simulink library "uavsimBlockset_ZagiUAS_externalForces"  (Simulink 8.0)
settings: Solver=ode45  StartTime=0.0  StopTime=10.0  RelTol=1e-3
libraries: uavsimBlockset_ServoHS55 x4, uavsimBlockset_Zagi_Aerandpropulsion x1, uavsimblockset_SixDOFKinematics x1
settings Model: Creator=mstolle  LastModifiedBy=j.bolting

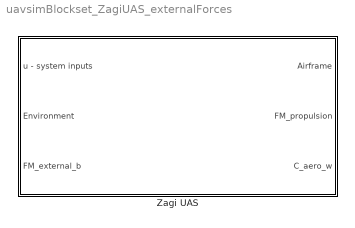
== system uavsimBlockset_ZagiUAS_externalForces ==
  Zagi UAS : Subsystem  mask{mask_zagi_phithetapsi0=[0 0 0]', mask_zagi_p0_ECEF_lla=[0 0 50]', mask_zagi_pqr0=[0 0 0]', mask_zagi_uvw0=[30 0 0]}
      mask prompts: mask_zagi_phithetapsi0 "Initial euler angles [rad]"; mask_zagi_p0_ECEF_lla "Initial position ECEF [rad rad m]"; mask_zagi_pqr0 "Initial body rotation rates [rad/s]"; mask_zagi_uvw0 "Initial velocity body frame [m/s]"
      mask Display: image(imread('images/zagi_slope.png'),[.3, .3, .4, .4])

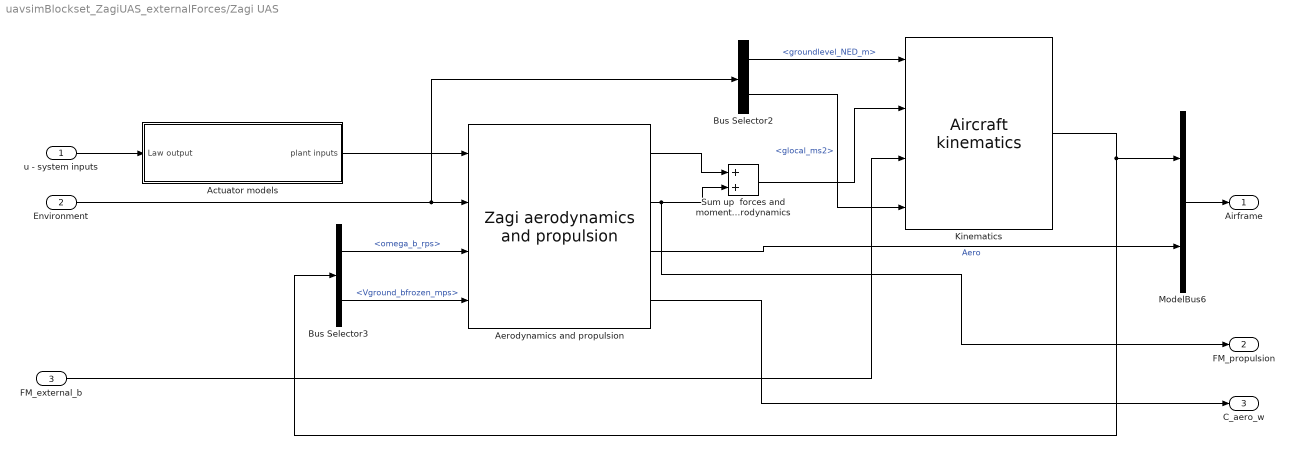
== system uavsimBlockset_ZagiUAS_externalForces/Zagi UAS ==
  u - system inputs : Inport  OutDataTypeStr=Bus: CMD
  Environment : Inport  Port=2  OutDataTypeStr=Bus: Environment
  FM_external_b : Inport  Port=3
  Actuator models : Subsystem
  Aerodynamics and propulsion : uavsimBlockset_Zagi_Aerandpropulsion/Zagi aerodynamics and propulsion  SystemSampleTime=-1
  Bus Selector2 : BusSelector  OutputSignals=groundlevel_NED_m,glocal_ms2
  Bus Selector3 : BusSelector  OutputSignals=RotationalVelocity.omega_b_rps,Velocity.Vground_bfrozen_mps
  Kinematics : uavsimblockset_SixDOFKinematics/Aircraft kinematics  mask_inertia=uavsim.zagi.inertiaTensor  mask_mass=uavsim.zagi.mass  mask_P0_ECEF_lla=mask_zagi_p0_ECEF_lla  mask_uvw0=mask_zagi_uvw0  mask_phithetapsi0=mask_zagi_phithetapsi0  mask_omega0=mask_zagi_pqr0
  ModelBus6 : BusCreator  Inputs=2  OutDataTypeStr=Bus: Airframe  NonVirtualBus=on
  Sum up  forces and moments of engine and aircraft aerodynamics : Sum
  Airframe : Outport  OutDataTypeStr=Bus: Airframe
  FM_propulsion : Outport  Port=2
  C_aero_w : Outport  Port=3
  wires:
  Kinematics/1 -> Bus Selector3/1, ModelBus6/1
  Bus Selector2/1 -> Kinematics/1  "<groundlevel_NED_m>"
  Bus Selector2/2 -> Kinematics/4  "<glocal_ms2>"
  u - system inputs/1 -> Actuator models/1(Law output)
  Bus Selector3/1 -> Aerodynamics and propulsion/3  "<omega_b_rps>"
  Bus Selector3/2 -> Aerodynamics and propulsion/4  "<Vground_bfrozen_mps>"
  ModelBus6/1 -> Airframe/1
  Aerodynamics and propulsion/3 -> ModelBus6/2  "Aero"
  Environment/1 -> Bus Selector2/1, Aerodynamics and propulsion/2
  Actuator models/1(plant inputs) -> Aerodynamics and propulsion/1
  FM_external_b/1 -> Kinematics/3
  Aerodynamics and propulsion/4 -> C_aero_w/1
  Aerodynamics and propulsion/1 -> Sum up  forces and moments of engine and aircraft aerodynamics/1
  Aerodynamics and propulsion/2 -> FM_propulsion/1, Sum up  forces and moments of engine and aircraft aerodynamics/2
  Sum up  forces and moments of engine and aircraft aerodynamics/1 -> Kinematics/2

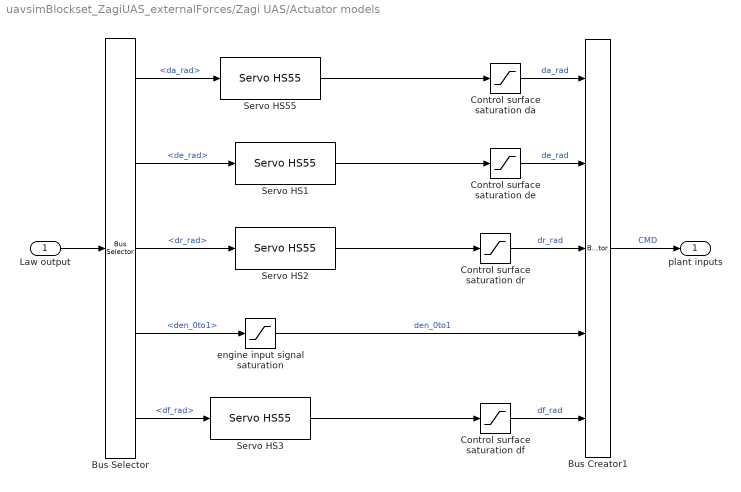
== system uavsimBlockset_ZagiUAS_externalForces/Zagi UAS/Actuator models ==
  Law output : Inport  OutDataTypeStr=Bus: CMD
  Bus Creator1 : BusCreator  Inputs=5  OutDataTypeStr=Bus: CMD  NonVirtualBus=on
  Bus Selector : BusSelector  OutputSignals=da_rad,de_rad,dr_rad,den_0to1,df_rad
  Control surface saturation da : Saturate  UpperLimit=deg2rad(45)  LowerLimit=deg2rad(-45)
  Control surface saturation de : Saturate  UpperLimit=deg2rad(45)  LowerLimit=deg2rad(-45)
  Control surface saturation df : Saturate  UpperLimit=deg2rad(45)  LowerLimit=deg2rad(-45)
  Control surface saturation dr : Saturate  UpperLimit=deg2rad(45)  LowerLimit=deg2rad(-45)
  Servo HS{1..3,55} (4 alike) : uavsimBlockset_ServoHS55/Servo HS55
  engine input signal saturation : Saturate  UpperLimit=1  LowerLimit=0
  plant inputs : Outport  OutDataTypeStr=Bus: CMD
  wires:
  Servo HS2/1 -> Control surface saturation dr/1
  Servo HS1/1 -> Control surface saturation de/1
  Servo HS55/1 -> Control surface saturation da/1
  Control surface saturation da/1 -> Bus Creator1/1  "da_rad"
  Control surface saturation de/1 -> Bus Creator1/2  "de_rad"
  Control surface saturation dr/1 -> Bus Creator1/3  "dr_rad"
  Bus Selector/1 -> Servo HS55/1  "<da_rad>"
  Bus Selector/2 -> Servo HS1/1  "<de_rad>"
  Bus Selector/3 -> Servo HS2/1  "<dr_rad>"
  Bus Selector/4 -> engine input signal saturation/1  "<den_0to1>"
  Law output/1 -> Bus Selector/1
  engine input signal saturation/1 -> Bus Creator1/4  "den_0to1"
  Bus Creator1/1 -> plant inputs/1  "CMD"
  Bus Selector/5 -> Servo HS3/1  "<df_rad>"
  Servo HS3/1 -> Control surface saturation df/1
  Control surface saturation df/1 -> Bus Creator1/5  "df_rad"
